simulink model "JointModel"  (R2024a)
settings: Solver=FixedStepAuto  StartTime=0.0  StopTime=8  FixedStep=1e-4  RelTol=1e-3
values from neighbouring files (symbols this model uses):
  CurrKi = 8.0    [JointData.sldd]
  CurrKp = 0.35    [JointData.sldd]
  flux = 0.00325    [JointData.sldd]
  Pn = 11.0    [JointData.sldd]
  Udc = 12.0    [JointData.sldd]
undefined symbols (not defined in the file or in its folder): curr_d_ki, curr_d_kp, curr_q_ki, curr_q_kp, DiscIntNeverNeededParam
libraries: slpidlib x2, mcbplantlib x1, autolibpmsmexterior x1, simulink x1
settings Model: DataDictionary=JointData.sldd  Creator=senki  LastModifiedBy=senki
settings OptimizationCC: DefaultParameterBehavior=Inlined  UseDivisionForNetSlopeComputation=on  GainParamInheritBuiltInType=on  UseFloatMulNetSlope=on  InlineInvariantSignals=on  PassReuseOutputArgsAs=Individual arguments  ZeroExternalMemoryAtStartup=off  ZeroInternalMemoryAtStartup=off  NoFixptDivByZeroProtection=on  EfficientFloat2IntCast=on  LifeSpan=1  OptimizeBlockOrder=speed  DifferentSizesBufferReuse=on  EfficientTunableParamExpr=on
settings DebuggingCC: ParameterTunabilityLossMsg=error
settings HardwareCC: ProdBitPerPointer=32  ProdBitPerSizeT=32  ProdBitPerPtrDiffT=32  ProdLargestAtomicInteger=Long  ProdLargestAtomicFloat=Double  ProdWordSize=32  ProdLongLongMode=on  ProdHWDeviceType=ARM Compatible->ARM Cortex-M
settings SFSimCC: MATLABDynamicMemAlloc=off
settings RTWCC: Description=Embedded Coder  SystemTargetFile=ert.tlc  TemplateMakefile=ert_default_tmf  GenerateReport=on  LaunchReport=on
settings CodeAppCC: ForceParamTrailComments=on  IgnoreCustomStorageClasses=off  OperatorAnnotations=on  SimulinkDataObjDesc=on  SFDataObjDesc=on  CustomSymbolStrGlobalVar=rt$N$M  CustomSymbolStrType=$N$M  CustomSymbolStrFcn=$N$M$F  CustomSymbolStrMacro=$N$M  InsertBlockDesc=on
settings ERTTargetCC: TargetLangStandard=C99 (ISO)  CodeReplacementLibrary=ARM Cortex-M  GenerateSampleERTMain=on  IncludeMdlTerminateFcn=off  CombineSignalStateStructs=on  SupportComplex=off  SupportNonInlinedSFcns=on  InlinedParameterPlacement=NonHierarchical  ERTCustomFileTemplate=example_file_process.tlc  ERTFilePackagingFormat=CompactWithDataFile

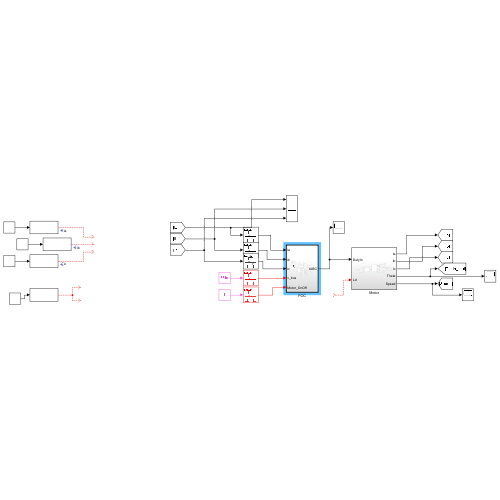
[thumbnail: Simulink's stored preview of the top-level diagram]
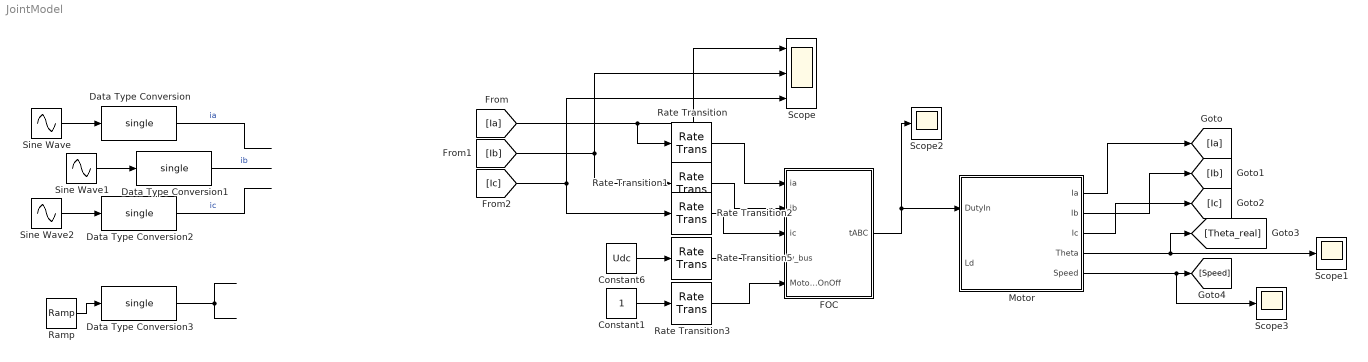
== system JointModel ==
  Constant1 : Constant  OutDataTypeStr=single
  Constant6 : Constant  Value=Udc  OutDataTypeStr=single
  Data Type Conversion{,1..3} (4 alike) : DataTypeConversion  OutDataTypeStr=single  SaturateOnIntegerOverflow=off  RndMeth=Floor
  FOC : Subsystem  TreatAsAtomicUnit=on
  Motor : Subsystem
  Ramp : simulink/Sources/Ramp  slope=502.6544  start=0  InitialOutput=0
  Rate Transition{,1..3,5} (5 alike) : RateTransition
  Scope : Scope  NumInputPorts=3
  Scope1 : Scope
  Scope2 : Scope
  Scope3 : Scope
  Sine Wave : Sin  Amplitude=5  Frequency=502.6544  SampleTime=1e-4
  Sine Wave1 : Sin  Amplitude=5  Frequency=502.6544  Phase=-2*pi/3  SampleTime=1e-4
  Sine Wave2 : Sin  Amplitude=5  Frequency=502.6544  Phase=-4*pi/3  SampleTime=1e-4
  wires:
  Motor/1(Ia) -> [Ia]
  Motor/2(Ib) -> [Ib]
  Motor/3(Ic) -> [Ic]
  Motor/4(Theta) -> [Theta_real], Scope1/1
  Data Type Conversion3/1 -> ?
  Sine Wave1/1 -> Data Type Conversion1/1
  Data Type Conversion2/1 -> ?  "ic"
  Ramp/1 -> Data Type Conversion3/1
  Sine Wave2/1 -> Data Type Conversion2/1
  Data Type Conversion/1 -> ?  "ia"
  Sine Wave/1 -> Data Type Conversion/1
  Data Type Conversion1/1 -> ?  "ib"
  [Ia] -> Scope/1, Rate Transition/1
  [Ib] -> Rate Transition1/1, Scope/2
  [Ic] -> Rate Transition2/1, Scope/3
  FOC/1(tABC) -> Scope2/1, Motor/1(DutyIn)
  Motor/5(Speed) -> Scope3/1, [Speed]
  ? -> Motor/2(Ld)
  Rate Transition/1 -> FOC/1(ia)
  Rate Transition1/1 -> FOC/2(ib)
  Rate Transition2/1 -> FOC/3(ic)
  Constant6/1 -> Rate Transition5/1
  Rate Transition5/1 -> FOC/4(v_bus)
  Constant1/1 -> Rate Transition3/1
  Rate Transition3/1 -> FOC/5(Motor_OnOff)

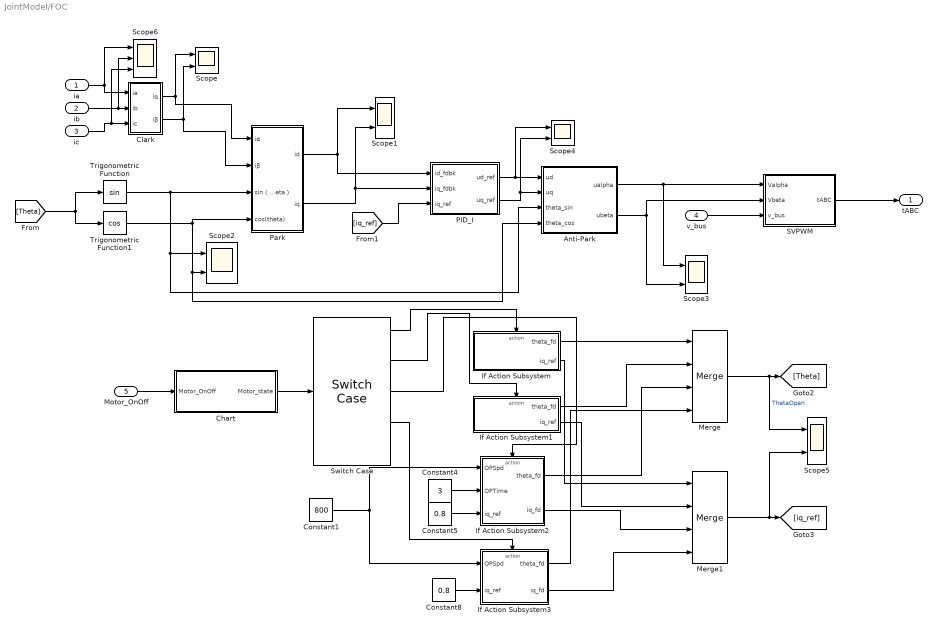
== system JointModel/FOC ==
  ia : Inport
  ib : Inport  Port=2
  ic : Inport  Port=3
  v_bus : Inport  Port=4  OutDataTypeStr=single
  Motor_OnOff : Inport  Port=5
  Anti-Park : Subsystem
  Chart : Stateflow chart  TreatAsAtomicUnit=on
  Clark : Subsystem
  Constant1 : Constant  Value=800  OutDataTypeStr=single
  Constant4 : Constant  Value=3  OutDataTypeStr=single
  Constant5 : Constant  Value=0.8  OutDataTypeStr=single
  Constant8 : Constant  Value=0.8  OutDataTypeStr=single
  If Action Subsystem : Subsystem  TreatAsAtomicUnit=on
  If Action Subsystem1 : Subsystem  TreatAsAtomicUnit=on
  If Action Subsystem2 : Subsystem  TreatAsAtomicUnit=on
  If Action Subsystem3 : Subsystem  TreatAsAtomicUnit=on
  Merge : Merge  Inputs=4
  Merge1 : Merge  Inputs=4
  PID_I : Subsystem
  Park : Subsystem
  SVPWM : Subsystem
  Scope{,1..5} (6 alike) : Scope  NumInputPorts=2
  Scope6 : Scope  NumInputPorts=3
  Switch Case : SwitchCase  CaseConditions={1,2,3,4}
  Trigonometric Function : Trigonometry
  Trigonometric Function1 : Trigonometry  Operator=cos
  tABC : Outport
  wires:
  Clark/2(iβ) -> Scope/2, Park/2(iβ)
  ic/1 -> Clark/3(ic), Scope6/3
  Anti-Park/1(ualpha) -> Scope3/1, SVPWM/1(Valpha)
  Park/2(iq) -> PID_I/2(iq_fdbk), Scope1/2
  Clark/1(iα) -> Scope/1, Park/1(iα)
  v_bus/1 -> SVPWM/3(v_bus)
  ia/1 -> Scope6/1, Clark/1(ia)
  Trigonometric Function/1 -> Scope2/1, Anti-Park/3(theta_sin), Park/3(sin（theta）)
  Trigonometric Function1/1 -> Anti-Park/4(theta_cos), Scope2/2, Park/4(cos(theta))
  Anti-Park/2(ubeta) -> Scope3/2, SVPWM/2(Vbeta)
  Park/1(id) -> PID_I/1(id_fdbk), Scope1/1
  PID_I/1(ud_ref) -> Anti-Park/1(ud), Scope4/1
  PID_I/2(uq_ref) -> Anti-Park/2(uq), Scope4/2
  ib/1 -> Scope6/2, Clark/2(ib)
  SVPWM/1(tABC) -> tABC/1
  Motor_OnOff/1 -> Chart/1(Motor_OnOff)
  Chart/1(Motor_state) -> Switch Case/1
  If Action Subsystem/2(iq_ref) -> Merge1/1
  Merge/1 -> Scope5/1, [Theta]  "ThetaOpen"
  If Action Subsystem1/2(iq_ref) -> Merge1/2
  Constant5/1 -> If Action Subsystem2/3(iq_ref)
  Merge1/1 -> Scope5/2, [iq_ref]
  If Action Subsystem3/1(theta_fd) -> Merge/4
  If Action Subsystem/1(theta_fd) -> Merge/1
  Constant4/1 -> If Action Subsystem2/2(OPTime)
  If Action Subsystem1/1(theta_fd) -> Merge/2
  If Action Subsystem2/2(iq_fd) -> Merge1/3
  Constant8/1 -> If Action Subsystem3/2(iq_ref)
  If Action Subsystem2/1(theta_fd) -> Merge/3
  If Action Subsystem3/2(iq_fd) -> Merge1/4
  Constant1/1 -> If Action Subsystem2/1(OPSpd), If Action Subsystem3/1(OPSpd)
  [Theta] -> Trigonometric Function1/1, Trigonometric Function/1
  [iq_ref] -> PID_I/3(iq_ref)
  Switch Case/1 -> If Action Subsystem/Action
  Switch Case/2 -> If Action Subsystem1/Action
  Switch Case/3 -> If Action Subsystem2/Action
  Switch Case/4 -> If Action Subsystem3/Action

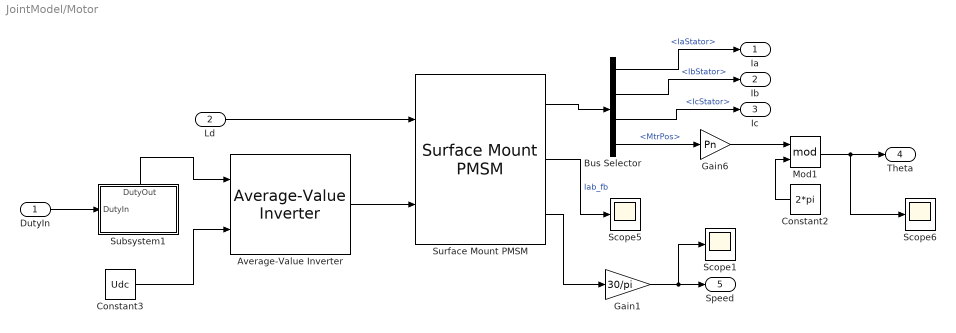
== system JointModel/Motor ==
  DutyIn : Inport
  Ld : Inport  Port=2
  Average-Value Inverter : mcbplantlib/Average-Value Inverter
  Bus Selector : BusSelector  OutputSignals=IaStator,IbStator,IcStator,MtrPos
  Constant2 : Constant  Value=2*pi  OutDataTypeStr=single
  Constant3 : Constant  Value=Udc
  Gain1 : Gain  Gain=30/pi  OutDataTypeStr=single
  Gain6 : Gain  Gain=Pn  OutDataTypeStr=single
  Mod1 : Math  Operator=mod  OutputSignalType=real
  Scope1 : Scope
  Scope5 : Scope
  Scope6 : Scope
  Subsystem1 : Subsystem
      settings: PortSchema="{\"entries\":[{\"content\":{\"sides\":[{\"content\":{\"connectorIds\":[\"In1\"]},\"type\":\"ConnectorPlacement.EquallySpacedRectSide\",\"uuid\":\"8ccc51de-fa2a-4900-80a3-4cdf9aa76f01\"},{\"content\":{\"connectorIds\":[],\"side\":\"RIGHT\"},\"type\":\"ConnectorPlacement.EquallySpacedRectSide\",\"uuid\":\"32c06e0d-3f1d-4948-af96-e310e54308a0\"},{\"content\":{\"connectorIds\":[\"Out1\"],\"side\":\"TOP\"},\"type\":\"ConnectorPlacement.EquallySpacedRectSide\",\"uuid\":\"a9066067-2c54-42a8-b4d7-fb86ac71b860\"}]},\"type\":\"ConnectorPlacement.EquallySpacedConnector\",\"uuid\":\"e4576975-acad-4e16-822f-2c2e7f23d7a7\"}],\"packageUris\":[\"http://schema.mathworks.com/mf0/Connector/R2020b\"],\"version\":\"1.0\"}"
  Surface Mount PMSM : autolibpmsmexterior/Surface Mount PMSM  port_config=Torque  sim_type=Discrete  Ts=1e-4  P=Pn  Rs=Rs  Ldq_=L  KConstText=Permanent flux linkage constant (lambda_pm):  lambda_pm=flux  Ke=0.0059268  Kt=0.061  mechanical=[5e-5, 1e-5, 0]  idq0=[0 0]  theta_init=4/5  omega_init=0  KConst=flux  lambda_pm_calc=flux  RefBlkName='autolibpmsmexterior/Surface Mount PMSM'  aMode=5  Ldq="[0.0017      0.0017]"
  Ia : Outport
  Ib : Outport  Port=2
  Ic : Outport  Port=3
  Theta : Outport  Port=4
  Speed : Outport  Port=5
  wires:
  Surface Mount PMSM/2 -> Scope5/1  "Iab_fb"
  Bus Selector/1 -> Ia/1  "<IaStator>"
  Surface Mount PMSM/1 -> Bus Selector/1
  Surface Mount PMSM/3 -> Gain1/1
  Bus Selector/3 -> Ic/1  "<IcStator>"
  Bus Selector/2 -> Ib/1  "<IbStator>"
  Gain6/1 -> Mod1/1
  Bus Selector/4 -> Gain6/1  "<MtrPos>"
  Constant3/1 -> Average-Value Inverter/2
  Constant2/1 -> Mod1/2
  Mod1/1 -> Theta/1, Scope6/1
  Subsystem1/1(DutyOut) -> Average-Value Inverter/1
  Average-Value Inverter/1 -> Surface Mount PMSM/2
  DutyIn/1 -> Subsystem1/1(DutyIn)
  Ld/1 -> Surface Mount PMSM/1
  Gain1/1 -> Scope1/1, Speed/1

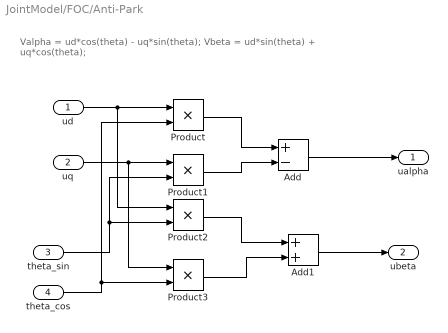
== system JointModel/FOC/Anti-Park ==
  note: Valpha = ud*cos(theta) - uq*sin(theta);
      | Vbeta = ud*sin(theta) + uq*cos(theta);
  ud : Inport
  uq : Inport  Port=2
  theta_sin : Inport  Port=3
  theta_cos : Inport  Port=4
  Add : Sum  Inputs=+-
  Add1 : Sum
  Product{,1..3} (4 alike) : Product
  ualpha : Outport  OutDataTypeStr=single
  ubeta : Outport  Port=2  OutDataTypeStr=single
  wires:
  Product/1 -> Add/1
  Product2/1 -> Add1/1
  uq/1 -> Product3/1, Product1/1
  Product3/1 -> Add1/2
  Product1/1 -> Add/2
  theta_cos/1 -> Product/2, Product3/2
  Add1/1 -> ubeta/1
  Add/1 -> ualpha/1
  theta_sin/1 -> Product2/2, Product1/2
  ud/1 -> Product2/1, Product/1

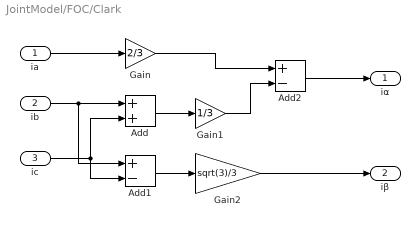
== system JointModel/FOC/Clark ==
  ia : Inport
  ib : Inport  Port=2
  ic : Inport  Port=3
  Add : Sum
  Add1 : Sum  Inputs=+-
  Add2 : Sum  Inputs=+-
  Gain : Gain  Gain=2/3
  Gain1 : Gain  Gain=1/3
  Gain2 : Gain  Gain=sqrt(3)/3
  iα : Outport
  iβ : Outport  Port=2
  wires:
  Add2/1 -> iα/1
  ib/1 -> Add/1, Add1/1
  ic/1 -> Add1/2, Add/2
  ia/1 -> Gain/1
  Gain1/1 -> Add2/2
  Gain/1 -> Add2/1
  Add1/1 -> Gain2/1
  Gain2/1 -> iβ/1
  Add/1 -> Gain1/1

== system JointModel/FOC/If Action Subsystem ==
  Action Port : ActionPort  ActionPortLabel=case [ 1 ]:
  Constant : Constant  Value=0  OutDataTypeStr=single
  Constant1 : Constant  Value=0  OutDataTypeStr=single
  theta_fd : Outport
  iq_ref : Outport  Port=2
  wires:
  Constant1/1 -> iq_ref/1
  Constant/1 -> theta_fd/1

== system JointModel/FOC/If Action Subsystem1 ==
  Action Port : ActionPort  ActionPortLabel=case [ 2 ]:
  Constant : Constant  Value=0  OutDataTypeStr=single
  Constant1 : Constant  Value=2  OutDataTypeStr=single
  theta_fd : Outport
  iq_ref : Outport  Port=2
  wires:
  Constant1/1 -> iq_ref/1
  Constant/1 -> theta_fd/1

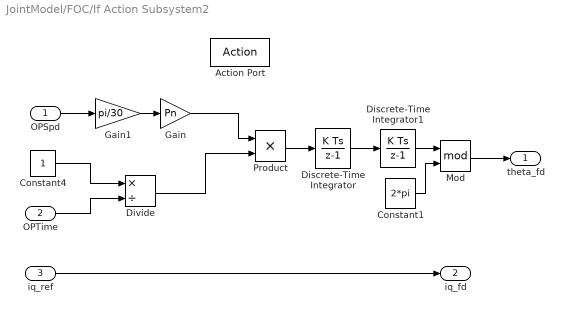
== system JointModel/FOC/If Action Subsystem2 ==
  OPSpd : Inport  OutDataTypeStr=single  PortDimensions=1
  OPTime : Inport  Port=2  OutDataTypeStr=single  PortDimensions=1
  iq_ref : Inport  Port=3
  Action Port : ActionPort  ActionPortLabel=case [ 3 ]:
  Constant1 : Constant  Value=2*pi  OutDataTypeStr=single
  Constant4 : Constant  OutDataTypeStr=single
  Discrete-Time Integrator : DiscreteIntegrator  SampleTime=-1  ICPrevOutput=DiscIntNeverNeededParam  ICPrevScaledInput=DiscIntNeverNeededParam
  Discrete-Time Integrator1 : DiscreteIntegrator  SampleTime=-1  ICPrevOutput=DiscIntNeverNeededParam  ICPrevScaledInput=DiscIntNeverNeededParam
  Divide : Product  Inputs=*/  OutDataTypeStr=single
  Gain : Gain  Gain=Pn
  Gain1 : Gain  Gain=pi/30  OutDataTypeStr=single
  Mod : Math  Operator=mod
  Product : Product  OutDataTypeStr=single
  theta_fd : Outport
  iq_fd : Outport  Port=2
  wires:
  iq_ref/1 -> iq_fd/1
  Constant4/1 -> Divide/1
  Constant1/1 -> Mod/2
  Discrete-Time Integrator1/1 -> Mod/1
  Gain1/1 -> Gain/1
  Divide/1 -> Product/2
  Discrete-Time Integrator/1 -> Discrete-Time Integrator1/1
  Mod/1 -> theta_fd/1
  Gain/1 -> Product/1
  Product/1 -> Discrete-Time Integrator/1
  OPSpd/1 -> Gain1/1
  OPTime/1 -> Divide/2

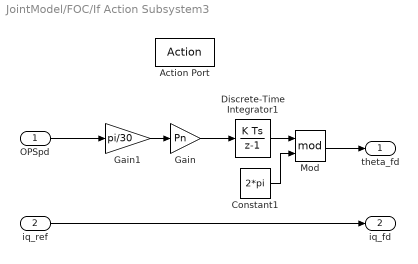
== system JointModel/FOC/If Action Subsystem3 ==
  OPSpd : Inport  OutDataTypeStr=single  PortDimensions=1
  iq_ref : Inport  Port=2
  Action Port : ActionPort  ActionPortLabel=case [ 4 ]:
  Constant1 : Constant  Value=2*pi  OutDataTypeStr=single
  Discrete-Time Integrator1 : DiscreteIntegrator  SampleTime=-1  ICPrevOutput=DiscIntNeverNeededParam  ICPrevScaledInput=DiscIntNeverNeededParam
  Gain : Gain  Gain=Pn
  Gain1 : Gain  Gain=pi/30  OutDataTypeStr=single
  Mod : Math  Operator=mod
  theta_fd : Outport
  iq_fd : Outport  Port=2
  wires:
  iq_ref/1 -> iq_fd/1
  OPSpd/1 -> Gain1/1
  Discrete-Time Integrator1/1 -> Mod/1
  Constant1/1 -> Mod/2
  Gain/1 -> Discrete-Time Integrator1/1
  Gain1/1 -> Gain/1
  Mod/1 -> theta_fd/1

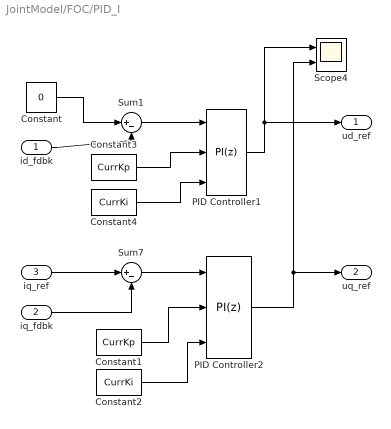
== system JointModel/FOC/PID_I ==
  id_fdbk : Inport  OutDataTypeStr=single
  iq_fdbk : Inport  Port=2  OutDataTypeStr=single
  iq_ref : Inport  Port=3  OutDataTypeStr=single
  Constant : Constant  Value=0  OutDataTypeStr=single
  Constant1 : Constant  Value=CurrKp  OutDataTypeStr=single
  Constant2 : Constant  Value=CurrKi  OutDataTypeStr=single
  Constant3 : Constant  Value=CurrKp  OutDataTypeStr=single
  Constant4 : Constant  Value=CurrKi  OutDataTypeStr=single
  PID Controller1 : slpidlib/PID Controller  Controller=PI  Form=Parallel  TimeDomain=Discrete-time  UseExternalTs=off  SampleTime=-1  IntegratorMethod=Forward Euler  FilterMethod=Forward Euler  ControllerParametersSource=external  P=curr_d_kp  I=curr_d_ki  UseKiTs=off  D=0  UseExternalDerivativeSource=off  N=100  UseFilter=on  TunerSelectOption=Transfer Function Based (PID Tuner App)  InitialConditionSource=internal  InitialConditionForIntegrator=0  InitialConditionForFilter=0  DifferentiatorICPrevScaledInput=0  ExternalReset=none  TrackingMode=off  Kt=1  LimitOutput=on  SatLimitsSource=internal  UpperSaturationLimit=12*0.9/sqrt(3)  LowerSaturationLimit=-12*0.9/sqrt(3)  LinearizeAsGain=on  AntiWindupMode=clamping  Kb=1  LimitIntegrator=off  UpperIntegratorSaturationLimit=inf  LowerIntegratorSaturationLimit=-inf  PGainOutDataTypeStr=single  PProdOutDataTypeStr=single  POutMin=[]  POutMax=[]  IGainOutDataTypeStr=int16  IProdOutDataTypeStr=int16  IOutMin=[]  IOutMax=[]  DOutMin=[]  DOutMax=[]  NOutMin=[]  NOutMax=[]  SumOutDataTypeStr=single  SumOutMin=[]  SumOutMax=[]  SaturationOutDataTypeStr=single  SaturationOutMin=[]  SaturationOutMax=[]  PParamMin=[]  PParamMax=[]  IParamMin=[]  IParamMax=[]  DParamMin=[]  DParamMax=[]  NParamMin=[]  NParamMax=[]  KbParamMin=[]  KbParamMax=[]  KtParamMin=[]  KtParamMax=[]  KbOutMin=[]  KbOutMax=[]  KtOutMin=[]  KtOutMax=[]  IntegratorOutMin=[]  IntegratorOutMax=[]  FilterOutMin=[]  FilterOutMax=[]  SumI1OutMin=[]  SumI1OutMax=[]  SumI2OutMin=[]  SumI2OutMax=[]  SumI3OutMin=[]  SumI3OutMax=[]  SumI4OutMin=[]  SumI4OutMax=[]  SumDOutMin=[]  SumDOutMax=[]  DifferentiatorOutMin=[]  DifferentiatorOutMax=[]  FilterDiffOutCoefMin=[]  FilterDiffOutCoefMax=[]  ReciprocalOutMin=[]  ReciprocalOutMax=[]  SumDenOutMin=[]  SumDenOutMax=[]  SumNumOutMin=[]  SumNumOutMax=[]  DivideOutMin=[]  DivideOutMax=[]  UdiffTsProdOutMin=[]  UdiffTsProdOutMax=[]  NTsProdOutMin=[]  NTsProdOutMax=[]  UintegralTsProdOutMin=[]  UintegralTsProdOutMax=[]  UngainTsProdOutMin=[]  UngainTsProdOutMax=[]  ClampingZeroOutDataTypeStr=Inherit: Inherit via back propagation  ClampingZeroOutMin=[]  ClampingZeroOutMax=[]  FilterDenConstantOutDataTypeStr=Inherit: Inherit via back propagation  FilterDenConstantOutMin=[]  FilterDenConstantOutMax=[]  PCopyOutDataTypeStr=Inherit: Inherit via back propagation  PCopyOutMin=[]  PCopyOutMax=[]  NCopyOutDataTypeStr=Inherit: Inherit via back propagation  NCopyOutMin=[]  NCopyOutMax=[]  IntegratorContinuousStateAttributes=''  IntegratorStateMustResolveToSignalObject=off  IntegratorRTWStateStorageClass=Auto  FilterContinuousStateAttributes=''  FilterStateMustResolveToSignalObject=off  FilterRTWStateStorageClass=Auto  ParallelPVariant=ExternalParameters  IdealPVariant=Disabled  IVariant=ExternalParameters  DVariant=Disabled  IntegratorVariant=Discrete  SatVariant=Enabled  AWVariant=DiscClampingParallel  PCopyVariant=Disabled  TRVariant=Disabled  FdbkBlocksVariant=Forward  IdealPFdbkVariant=Disabled  SatFdbkVariant=Disabled  DerivativeFilterVariant=Disabled  NVariant=Disabled  NCopyVariant=Disabled_SignalSpec  FilterICVariant=Disabled  IntegratorICVariant=InternalICs  ExternalResetVariant=Disabled  TRSumVariant=Passthrough  SumFdbkVariant=Disabled  SumVariant=Sum_PI  TsampFilterVariant=InternalTs  TsampNgainVariant=Passthrough  TsampIntegralVariant=Disabled_SignalSpec  ExternalSaturationOutDataTypeStr=Inherit: Same as second input  DerivativeSourceVariant=Disabled
  PID Controller2 : slpidlib/PID Controller  Controller=PI  Form=Parallel  TimeDomain=Discrete-time  UseExternalTs=off  SampleTime=-1  IntegratorMethod=Forward Euler  FilterMethod=Forward Euler  ControllerParametersSource=external  P=curr_q_kp  I=curr_q_ki  UseKiTs=off  D=0  UseExternalDerivativeSource=off  N=100  UseFilter=on  TunerSelectOption=Transfer Function Based (PID Tuner App)  InitialConditionSource=internal  InitialConditionForIntegrator=0  InitialConditionForFilter=0  DifferentiatorICPrevScaledInput=0  ExternalReset=none  TrackingMode=off  Kt=1  LimitOutput=on  SatLimitsSource=internal  UpperSaturationLimit=12*0.9/sqrt(3)  LowerSaturationLimit=-12*0.9/sqrt(3)  LinearizeAsGain=on  AntiWindupMode=clamping  Kb=1  LimitIntegrator=off  UpperIntegratorSaturationLimit=inf  LowerIntegratorSaturationLimit=-inf  PGainOutDataTypeStr=single  PProdOutDataTypeStr=single  POutMin=[]  POutMax=[]  IGainOutDataTypeStr=single  IProdOutDataTypeStr=single  IOutMin=[]  IOutMax=[]  DOutMin=[]  DOutMax=[]  NOutMin=[]  NOutMax=[]  SumOutDataTypeStr=single  SumOutMin=[]  SumOutMax=[]  SaturationOutDataTypeStr=single  SaturationOutMin=[]  SaturationOutMax=[]  PParamMin=[]  PParamMax=[]  IParamMin=[]  IParamMax=[]  DParamMin=[]  DParamMax=[]  NParamMin=[]  NParamMax=[]  KbParamMin=[]  KbParamMax=[]  KtParamMin=[]  KtParamMax=[]  KbOutMin=[]  KbOutMax=[]  KtOutMin=[]  KtOutMax=[]  IntegratorOutMin=[]  IntegratorOutMax=[]  FilterOutMin=[]  FilterOutMax=[]  SumI1OutMin=[]  SumI1OutMax=[]  SumI2OutMin=[]  SumI2OutMax=[]  SumI3OutMin=[]  SumI3OutMax=[]  SumI4OutMin=[]  SumI4OutMax=[]  SumDOutMin=[]  SumDOutMax=[]  DifferentiatorOutMin=[]  DifferentiatorOutMax=[]  FilterDiffOutCoefMin=[]  FilterDiffOutCoefMax=[]  ReciprocalOutMin=[]  ReciprocalOutMax=[]  SumDenOutMin=[]  SumDenOutMax=[]  SumNumOutMin=[]  SumNumOutMax=[]  DivideOutMin=[]  DivideOutMax=[]  UdiffTsProdOutMin=[]  UdiffTsProdOutMax=[]  NTsProdOutMin=[]  NTsProdOutMax=[]  UintegralTsProdOutMin=[]  UintegralTsProdOutMax=[]  UngainTsProdOutMin=[]  UngainTsProdOutMax=[]  ClampingZeroOutDataTypeStr=Inherit: Inherit via back propagation  ClampingZeroOutMin=[]  ClampingZeroOutMax=[]  FilterDenConstantOutDataTypeStr=Inherit: Inherit via back propagation  FilterDenConstantOutMin=[]  FilterDenConstantOutMax=[]  PCopyOutDataTypeStr=Inherit: Inherit via back propagation  PCopyOutMin=[]  PCopyOutMax=[]  NCopyOutDataTypeStr=Inherit: Inherit via back propagation  NCopyOutMin=[]  NCopyOutMax=[]  IntegratorContinuousStateAttributes=''  IntegratorStateMustResolveToSignalObject=off  IntegratorRTWStateStorageClass=Auto  FilterContinuousStateAttributes=''  FilterStateMustResolveToSignalObject=off  FilterRTWStateStorageClass=Auto  ParallelPVariant=ExternalParameters  IdealPVariant=Disabled  IVariant=ExternalParameters  DVariant=Disabled  IntegratorVariant=Discrete  SatVariant=Enabled  AWVariant=DiscClampingParallel  PCopyVariant=Disabled  TRVariant=Disabled  FdbkBlocksVariant=Forward  IdealPFdbkVariant=Disabled  SatFdbkVariant=Disabled  DerivativeFilterVariant=Disabled  NVariant=Disabled  NCopyVariant=Disabled_SignalSpec  FilterICVariant=Disabled  IntegratorICVariant=InternalICs  ExternalResetVariant=Disabled  TRSumVariant=Passthrough  SumFdbkVariant=Disabled  SumVariant=Sum_PI  TsampFilterVariant=InternalTs  TsampNgainVariant=Passthrough  TsampIntegralVariant=Disabled_SignalSpec  ExternalSaturationOutDataTypeStr=Inherit: Same as second input  DerivativeSourceVariant=Disabled
  Scope4 : Scope  NumInputPorts=2
  Sum1 : Sum  Inputs=|+-  OutDataTypeStr=single  AccumDataTypeStr=single
  Sum7 : Sum  Inputs=|+-  OutDataTypeStr=single  AccumDataTypeStr=single
  ud_ref : Outport  OutDataTypeStr=single
  uq_ref : Outport  Port=2  OutDataTypeStr=single
  wires:
  PID Controller1/1 -> ud_ref/1, Scope4/1
  Constant1/1 -> PID Controller2/2
  PID Controller2/1 -> Scope4/2, uq_ref/1
  Constant4/1 -> PID Controller1/3
  Constant/1 -> Sum1/1
  Sum7/1 -> PID Controller2/1
  Constant2/1 -> PID Controller2/3
  Sum1/1 -> PID Controller1/1
  Constant3/1 -> PID Controller1/2
  id_fdbk/1 -> Sum1/2
  iq_fdbk/1 -> Sum7/2
  iq_ref/1 -> Sum7/1

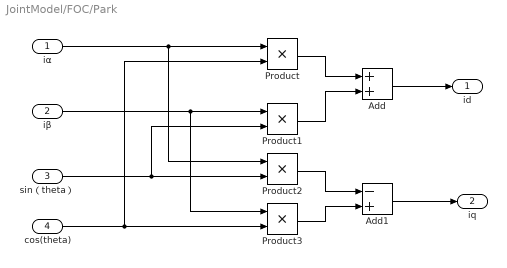
== system JointModel/FOC/Park ==
  iα : Inport
  iβ : Inport  Port=2
  sin（theta） : Inport  Port=3
  cos(theta) : Inport  Port=4
  Add : Sum  OutDataTypeStr=single  AccumDataTypeStr=single
  Add1 : Sum  Inputs=-+  OutDataTypeStr=single  AccumDataTypeStr=single
  Product{,1..3} (4 alike) : Product  OutDataTypeStr=single
  id : Outport  OutDataTypeStr=single
  iq : Outport  Port=2  OutDataTypeStr=single
  wires:
  sin（theta）/1 -> Product1/2, Product2/2
  iα/1 -> Product/1, Product2/1
  Product3/1 -> Add1/2
  Product1/1 -> Add/2
  Add/1 -> id/1
  iβ/1 -> Product3/1, Product1/1
  Product2/1 -> Add1/1
  Add1/1 -> iq/1
  cos(theta)/1 -> Product3/2, Product/2
  Product/1 -> Add/1

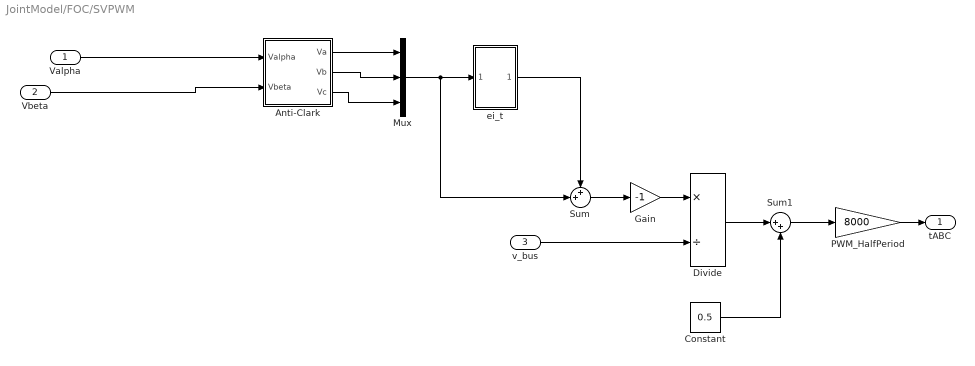
== system JointModel/FOC/SVPWM ==
  Valpha : Inport
  Vbeta : Inport  Port=2
  v_bus : Inport  Port=3  OutDataTypeStr=single
  Anti-Clark : Subsystem
  Constant : Constant  Value=0.5  OutDataTypeStr=single
  Divide : Product  Inputs=*/  OutDataTypeStr=single
  Gain : Gain  Gain=-1  OutDataTypeStr=single
  Mux : Mux  Inputs=3
  PWM_HalfPeriod : Gain  Gain=8000  OutDataTypeStr=single
  Sum : Sum  Inputs=++|  OutDataTypeStr=single
  Sum1 : Sum  Inputs=|++  OutDataTypeStr=single
  ei_t : Subsystem
  tABC : Outport  OutDataTypeStr=single
  wires:
  PWM_HalfPeriod/1 -> tABC/1
  Mux/1 -> Sum/2, ei_t/1(Vabc)
  Constant/1 -> Sum1/2
  Divide/1 -> Sum1/1
  Anti-Clark/1(Va) -> Mux/1
  Anti-Clark/2(Vb) -> Mux/2
  ei_t/1(ei_t) -> Sum/1
  Anti-Clark/3(Vc) -> Mux/3
  Sum1/1 -> PWM_HalfPeriod/1
  Sum/1 -> Gain/1
  Gain/1 -> Divide/1
  v_bus/1 -> Divide/2
  Vbeta/1 -> Anti-Clark/2(Vbeta)
  Valpha/1 -> Anti-Clark/1(Valpha)

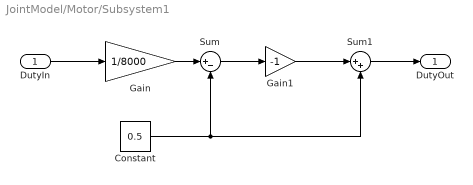
== system JointModel/Motor/Subsystem1 ==
  DutyIn : Inport
  Constant : Constant  Value=0.5  SampleTime=-1
  Gain : Gain  Gain=1/8000  ParamDataTypeStr=single
  Gain1 : Gain  Gain=-1
  Sum : Sum  Inputs=|+-
  Sum1 : Sum  Inputs=|++
  DutyOut : Outport
  wires:
  Sum/1 -> Gain1/1
  Constant/1 -> Sum1/2, Sum/2
  DutyIn/1 -> Gain/1
  Gain1/1 -> Sum1/1
  Sum1/1 -> DutyOut/1
  Gain/1 -> Sum/1

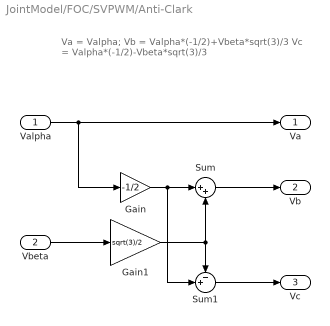
== system JointModel/FOC/SVPWM/Anti-Clark ==
  note: Va = Valpha;
      | Vb = Valpha*(-1/2)+Vbeta*sqrt(3)/3
      | Vc = Valpha*(-1/2)-Vbeta*sqrt(3)/3
  Valpha : Inport  OutDataTypeStr=single
  Vbeta : Inport  Port=2  OutDataTypeStr=single
  Gain : Gain  Gain=-1/2  OutDataTypeStr=single
  Gain1 : Gain  Gain=sqrt(3)/2  OutDataTypeStr=single
  Sum : Sum  Inputs=|++  OutDataTypeStr=single
  Sum1 : Sum  Inputs=-+|  OutDataTypeStr=single
  Va : Outport  OutDataTypeStr=single
  Vb : Outport  Port=2  OutDataTypeStr=single
  Vc : Outport  Port=3  OutDataTypeStr=single
  wires:
  Valpha/1 -> Va/1, Gain/1
  Vbeta/1 -> Gain1/1
  Gain1/1 -> Sum/2, Sum1/1
  Sum/1 -> Vb/1
  Sum1/1 -> Vc/1
  Gain/1 -> Sum1/2, Sum/1

== system JointModel/FOC/SVPWM/ei_t ==
  note: V0 = -1/2(Vmax+Vmin)
  Vabc : Inport  OutDataTypeStr=single
  Demux : Demux  Outputs=3
  Gain : Gain  Gain=-1/2  OutDataTypeStr=single
  Min : MinMax  Inputs=3  OutDataTypeStr=single
  Min1 : MinMax  Function=max  Inputs=3  OutDataTypeStr=single
  Sum : Sum  Inputs=|++  OutDataTypeStr=single
  ei_t : Outport  OutDataTypeStr=single
  wires:
  Demux/2 -> Min/2, Min1/2
  Vabc/1 -> Demux/1
  Min/1 -> Sum/1
  Demux/1 -> Min1/1, Min/1
  Demux/3 -> Min1/3, Min/3
  Gain/1 -> ei_t/1
  Min1/1 -> Sum/2
  Sum/1 -> Gain/1

== stateflow chart JointModel/FOC/Chart ==
  state IDLE
    en:
    du:
    Motor_state = 1;
  state AlignStage
    en:
    du:
    Motor_state = 2;
  state OpenStage
    en:
    du:
    Motor_state = 3;
  state RunStage
    en:
    du:
    Motor_state = 4;
  (default) -> IDLE
  IDLE -> AlignStage : [Motor_OnOff == 1]
  AlignStage -> OpenStage [order 1] : [after(1000,tick)]
  OpenStage -> RunStage [order 1] : [after(30000,tick)]
  OpenStage -> IDLE [order 2] : [Motor_OnOff == 0]
  AlignStage -> IDLE [order 2] : [Motor_OnOff == 0]
  RunStage -> IDLE : [Motor_OnOff == 0]
  data: Motor_OnOff input; Motor_state output
